simulink library "INP_DRVR_Prep"  (R2024b)
settings: Solver=VariableStepAuto  StartTime=0.0  StopTime=10.0  RelTol=1e-3
undefined symbols (not defined in the file): INP_c_TiSample_s, INP_DRVR_p_AngStWhlOfs_rad, INP_DRVR_p_AngStWhlSca_na, INP_DRVR_p_PosThrOfs_p100, INP_DRVR_p_PosThrSca_na, INP_p_TiTau_s
libraries: VUT_lib x4
settings Model: Creator=blatak  LastModifiedBy=blatak

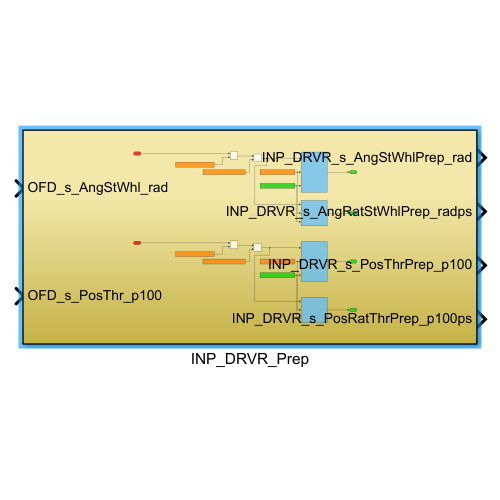
[thumbnail: Simulink's stored preview of the top-level diagram]
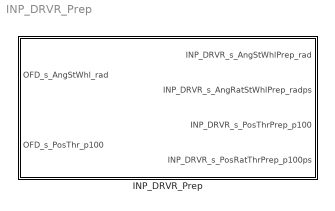
== system INP_DRVR_Prep ==
  INP_DRVR_Prep : Subsystem

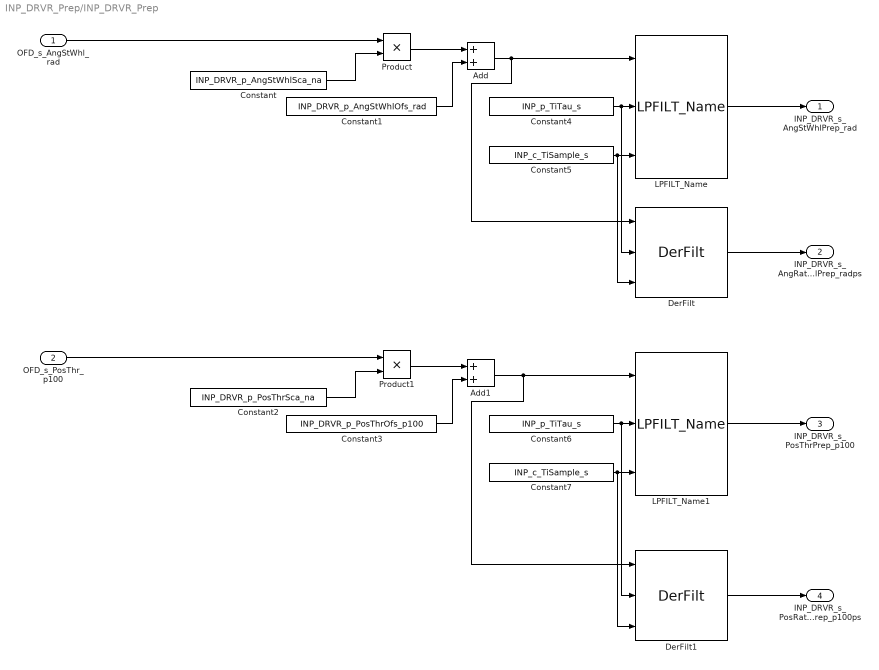
== system INP_DRVR_Prep/INP_DRVR_Prep ==
  OFD_s_AngStWhl_rad : Inport
  OFD_s_PosThr_p100 : Inport  Port=2
  Add : Sum
  Add1 : Sum
  Constant : Constant  Description=Scaling coefficient to recalculate the electric quantity to the physical one - longitudinal acceleration  Value=INP_DRVR_p_AngStWhlSca_na
  Constant1 : Constant  Description=Offset to recalculate the electric quantity to the physical one - longitudinal acceleration  Value=INP_DRVR_p_AngStWhlOfs_rad
  Constant2 : Constant  Description=Scaling coefficient to recalculate the electric quantity to the physical one - longitudinal acceleration  Value=INP_DRVR_p_PosThrSca_na
  Constant3 : Constant  Description=Offset to recalculate the electric quantity to the physical one - longitudinal acceleration  Value=INP_DRVR_p_PosThrOfs_p100
  Constant4 : Constant  Value=INP_p_TiTau_s
  Constant5 : Constant  Value=INP_c_TiSample_s
  Constant6 : Constant  Value=INP_p_TiTau_s
  Constant7 : Constant  Value=INP_c_TiSample_s
  DerFilt : VUT_lib/DerFilt  SystemSampleTime=-1  VariantActivationTime=update diagram  AllowFlexibleInterface=on  Latency=0  AutoFrameSizeCalculation=off
  DerFilt1 : VUT_lib/DerFilt  SystemSampleTime=-1  VariantActivationTime=update diagram  AllowFlexibleInterface=on  Latency=0  AutoFrameSizeCalculation=off
  LPFILT_Name : VUT_lib/LPFILT_Name  SystemSampleTime=-1  VariantActivationTime=update diagram  AllowFlexibleInterface=on  Latency=0  AutoFrameSizeCalculation=off
  LPFILT_Name1 : VUT_lib/LPFILT_Name  SystemSampleTime=-1  VariantActivationTime=update diagram  AllowFlexibleInterface=on  Latency=0  AutoFrameSizeCalculation=off
  Product : Product
  Product1 : Product
  INP_DRVR_s_AngStWhlPrep_rad : Outport
  INP_DRVR_s_AngRatStWhlPrep_radps : Outport  Port=2
  INP_DRVR_s_PosThrPrep_p100 : Outport  Port=3
  INP_DRVR_s_PosRatThrPrep_p100ps : Outport  Port=4
  wires:
  LPFILT_Name/1 -> INP_DRVR_s_AngStWhlPrep_rad/1
  OFD_s_PosThr_p100/1 -> Product1/1
  DerFilt1/1 -> INP_DRVR_s_PosRatThrPrep_p100ps/1
  Constant6/1 -> DerFilt1/2, LPFILT_Name1/2
  Constant4/1 -> DerFilt/2, LPFILT_Name/2
  DerFilt/1 -> INP_DRVR_s_AngRatStWhlPrep_radps/1
  Add/1 -> DerFilt/1, LPFILT_Name/1
  OFD_s_AngStWhl_rad/1 -> Product/1
  Constant/1 -> Product/2
  Constant7/1 -> DerFilt1/3, LPFILT_Name1/3
  Constant3/1 -> Add1/2
  Constant5/1 -> DerFilt/3, LPFILT_Name/3
  Add1/1 -> DerFilt1/1, LPFILT_Name1/1
  Constant2/1 -> Product1/2
  Product1/1 -> Add1/1
  LPFILT_Name1/1 -> INP_DRVR_s_PosThrPrep_p100/1
  Product/1 -> Add/1
  Constant1/1 -> Add/2
